simulink model "SentinelEciEcefTransformHarness"  (R2025a)
settings: Solver=ode4  StartTime=0.0  StopTime=890  FixedStep=10  RelTol=1e-3
undefined symbols (not defined in the file): IAU
libraries: aerolibtransform2 x1
settings Model: Creator=aocs-simulation  LastModifiedBy=juliankazmierski

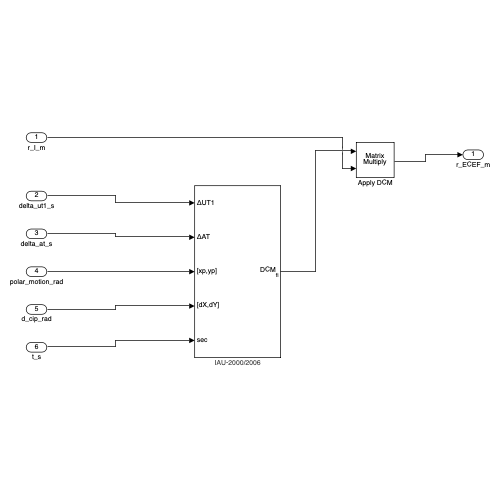
[thumbnail: Simulink's stored preview of the top-level diagram]
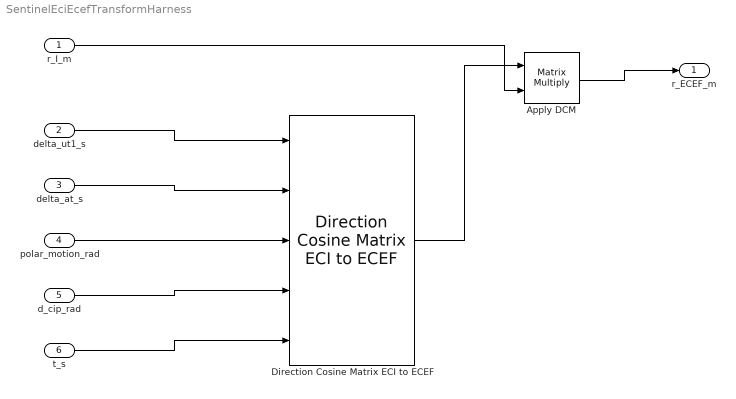
== system SentinelEciEcefTransformHarness ==
  r_I_m : Inport  OutDataTypeStr=double  PortDimensions=3
  delta_ut1_s : Inport  Port=2  OutDataTypeStr=double  PortDimensions=1
  delta_at_s : Inport  Port=3  OutDataTypeStr=double  PortDimensions=1
  polar_motion_rad : Inport  Port=4  OutDataTypeStr=double  PortDimensions=2
  d_cip_rad : Inport  Port=5  OutDataTypeStr=double  PortDimensions=2
  t_s : Inport  Port=6  OutDataTypeStr=double  PortDimensions=1
  Apply DCM : Product  Inputs=**  Multiplication=Matrix(*)
  Direction Cosine Matrix ECI to ECEF : aerolibtransform2/Direction Cosine Matrix ECI to ECEF  red=IAU-2000/2006  year=2024  month=January  day=1  hour=0  min=0  sec=2  deltaT=Sec  errorflag=Error  extraparamflag=on
      settings: AttributesFormatString=%<red>
  r_ECEF_m : Outport
  wires:
  delta_ut1_s/1 -> Direction Cosine Matrix ECI to ECEF/1
  delta_at_s/1 -> Direction Cosine Matrix ECI to ECEF/2
  polar_motion_rad/1 -> Direction Cosine Matrix ECI to ECEF/3
  d_cip_rad/1 -> Direction Cosine Matrix ECI to ECEF/4
  t_s/1 -> Direction Cosine Matrix ECI to ECEF/5
  Direction Cosine Matrix ECI to ECEF/1 -> Apply DCM/1
  r_I_m/1 -> Apply DCM/2
  Apply DCM/1 -> r_ECEF_m/1
